simulink model "Just_The_Electrical_model"  (R2016a)
settings: Solver=VariableStepAuto  StartTime=0.0  StopTime=10.0  RelTol=1e-3
values from neighbouring files (symbols this model uses):
  BT = {}    [Electrical_model_settings.m]
  btc = {}    [Electrical_model_settings.m]
  col = {}    [Electrical_model_settings.m]
  elc = {}    [Electrical_model_settings.m]
  ess = {}    [Electrical_model_settings.m]
  fcc = {}    [Electrical_model_settings.m]
  flex = {}    [Electrical_model_settings.m]
  systemBase = {}    [Electrical_model_settings.m]
  wf = {}    [Electrical_model_settings.m]
  wt1 = {}    [Electrical_model_settings.m]
  wt2 = wt1    [Electrical_model_settings.m]
  wt3 = wt1    [Electrical_model_settings.m]
undefined symbols (not defined in the file or in its folder): avr, D1, Delta, DiscIntNeverNeededParam, f2ctrl, governor, interface, Lf1, sm, Ts, Ts_phy, Ts_sim, u0
libraries: powerlib x69, pwrsysBasic x68, simulink_extras x37, pwrsysVICtrl x22, powerlib_meascontrol x19, simulink x8, pwrsysVSrc x5, pwrsysTransf x5, pwrsys-matlab x1
(part 3 of 4)

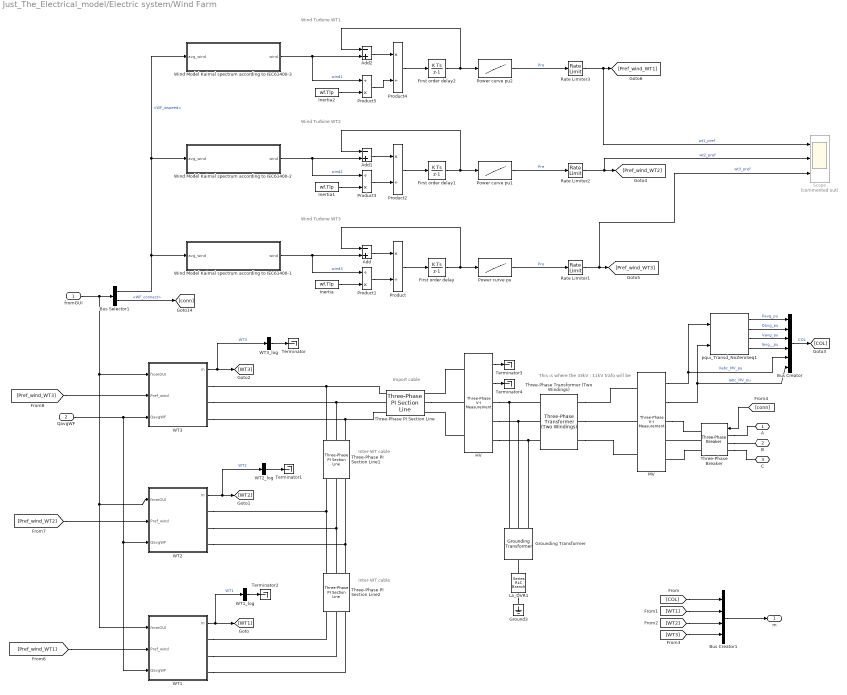
== system Just_The_Electrical_model/Electric system/Wind Farm ==
  note: Import cable
  note: This is where the 33kV : 11kV trafo will be
  note: Inter-WT cable
  note: Inter-WT cable
  note: Wind Turbine WT3
  note: Wind Turbine WT2
  note: Wind Turbine WT1
  fromGUI : Inport
  QavgWF : Inport  Port=2
  Add : Sum  Inputs=-+
  Add1 : Sum  Inputs=-+
  Add2 : Sum  Inputs=-+
  Bus Creator : BusCreator  Inputs=6
  Bus Creator1 : BusCreator  Inputs=4
  Bus Selector1 : BusSelector  OutputSignals=WF_wspeed,WF_connect
  First order delay : DiscreteIntegrator  gainval=1  SampleTime=Ts  ICPrevOutput=DiscIntNeverNeededParam  ICPrevScaledInput=DiscIntNeverNeededParam
  First order delay1 : DiscreteIntegrator  gainval=1  SampleTime=Ts  ICPrevOutput=DiscIntNeverNeededParam  ICPrevScaledInput=DiscIntNeverNeededParam
  First order delay2 : DiscreteIntegrator  gainval=1  SampleTime=Ts  ICPrevOutput=DiscIntNeverNeededParam  ICPrevScaledInput=DiscIntNeverNeededParam
  Ground3 : powerlib/Elements/Ground  LConnTagsString=a
  "Grounding Transformer " : powerlib/Elements/Grounding Transformer   UNITS=pu  NominalPower=[ col.Sn , systemBase.fn ]  NominalVoltage=systemBase.Vn  ZeroSequenceImpedance_pu=[0.025 0.75]  MagnetizationBranch_pu=[500 500]  ZeroSequenceImpedance_SI=[0.052083 589.05]  MagnetizationBranch_SI=[1041.7 3.927e+005]  Measurements=None
  HV : powerlib/Measurements/Three-Phase V-I Measurement  VoltageMeasurement=phase-to-ground  SetLabelV=off  LabelV=vgrid  Vpu=off  VpuLL=off  CurrentMeasurement=yes  SetLabelI=off  LabelI=igrid  Ipu=off  Pbase=sn  Vbase=uab  OutputType=Complex  PhasorSimulation=off  PSBequivalent=0
  Inertia : Constant  Value=wf.Tlp  SampleTime=-1
  Inertia1 : Constant  Value=wf.Tlp  SampleTime=-1
  Inertia2 : Constant  Value=wf.Tlp  SampleTime=-1
  La_DVR1 : powerlib/Elements/Series RLC Branch  LConnTagsString=__new0  RConnTagsString=__new0  BranchType=R  Resistance=250  Inductance=Lf1  SetiL0=off  InitialCurrent=0  Capacitance=1.0  Setx0=off  InitialVoltage=0  Measurements=None
  MV : powerlib/Measurements/Three-Phase V-I Measurement  VoltageMeasurement=phase-to-ground  SetLabelV=off  LabelV=vgrid  Vpu=off  VpuLL=off  CurrentMeasurement=yes  SetLabelI=off  LabelI=igrid  Ipu=off  Pbase=sn  Vbase=uab  OutputType=Complex  PhasorSimulation=off  PSBequivalent=0
  Power curve pu : Lookup  InputValues=wf.pcurve.wind  Table=wf.pcurve.power
  Power curve pu1 : Lookup  InputValues=wf.pcurve.wind  Table=wf.pcurve.power
  Power curve pu2 : Lookup  InputValues=wf.pcurve.wind  Table=wf.pcurve.power
  Product : Product  Inputs=*/
  Product1 : Product  Inputs=/*
  Product2 : Product  Inputs=*/
  Product3 : Product  Inputs=/*
  Product4 : Product  Inputs=*/
  Product5 : Product  Inputs=/*
  Rate Limiter1 : RateLimiter  RisingSlewLimit=100  FallingSlewLimit=-100  SampleTimeMode=inherited
  Rate Limiter2 : RateLimiter  RisingSlewLimit=100  FallingSlewLimit=-100  SampleTimeMode=inherited
  Rate Limiter3 : RateLimiter  RisingSlewLimit=100  FallingSlewLimit=-100  SampleTimeMode=inherited
  Scope : Scope  Commented=on  NumInputPorts=3
  Terminator{,1..4} (5 alike) : Terminator
  Three-Phase PI Section Line : powerlib/Elements/Three-Phase PI Section Line  LConnTagsString=a|b|c  RConnTagsString=A|B|C  Frequency=systemBase.fn  Resistances=[ col.Cable.Rpos col.Cable.Rzero]  Inductances=[ col.Cable.Lpos col.Cable.Lzero]  Capacitances=[col.Cable.Cpos col.Cable.Czero]  Length=col.Cable.Limport
  Three-Phase PI Section Line1 : powerlib/Elements/Three-Phase PI Section Line  LConnTagsString=a|b|c  RConnTagsString=A|B|C  Frequency=systemBase.fn  Resistances=[ col.Cable.Rpos col.Cable.Rzero]  Inductances=[ col.Cable.Lpos col.Cable.Lzero]  Capacitances=[col.Cable.Cpos col.Cable.Czero]  Length=col.Cable.LinterWT
  Three-Phase PI Section Line2 : powerlib/Elements/Three-Phase PI Section Line  LConnTagsString=a|b|c  RConnTagsString=A|B|C  Frequency=systemBase.fn  Resistances=[ col.Cable.Rpos col.Cable.Rzero]  Inductances=[ col.Cable.Lpos col.Cable.Lzero]  Capacitances=[col.Cable.Cpos col.Cable.Czero]  Length=col.Cable.LinterWT
  Three-Phase Transformer (Two Windings) : powerlib/Elements/Three-Phase Transformer (Two Windings)  Winding1Connection=Y  Winding2Connection=Delta (D1)  CoreType=Three-limb core (core-type)  SetSaturation=off  Hysteresis=off  DataFile='hysteresis'  SetInitialFlux=off  Measurements=None  UNITS=pu  NominalPower=[ col.Sn , systemBase.fn ]  Winding1=[ systemBase.Vn , col.Trafo.rsc/2 , col.Trafo.xsc/2 ]  Winding2=[ col.Un , col.Trafo.rsc/2 , col.Trafo.xsc/2 ]  Rm=500  Lm=500  L0=0.5  Saturation=[ 0,0 ; 0.0024,1.2 ; 1.0,1.52 ]  InitialFluxes=[0 0 0]  MoreParameters=off  BreakLoop=off  DataType=off  TransfoNumber=1
  Three-Phase Breaker : powerlib/Elements/Three-Phase Breaker  InitialState=closed  SwitchA=on  SwitchB=on  SwitchC=on  SwitchTimes="[1/60  5/60]"  External=on  BreakerResistance=0.01  SnubberResistance=1e6  SnubberCapacitance=1e9  Measurements=None
  WT1 : Subsystem
  WT1_log : BusSelector  OutputSignals=Pavg_pu,Qavg_pu,Vavg_pu,Vdc_pu,Idc_pu  OutputAsBus=on
  WT2 : Subsystem
  WT2_log : BusSelector  OutputSignals=Pavg_pu,Qavg_pu,Vavg_pu,Vdc_pu,Idc_pu  OutputAsBus=on
  WT3 : Subsystem
  WT3_log : BusSelector  OutputSignals=Pavg_pu,Qavg_pu,Vavg_pu,Vdc_pu,Idc_pu  OutputAsBus=on
  Wind Model Kaimal spectrum according to IEC61400-1 : Subsystem  TreatAsAtomicUnit=on  mask(Wind Model using Simulink Band-limited white noise generator){D_rotor=wf.Rdiam, L=wf.Lmm, turb_int=wf.Turb, T_sample=1/systemBase.fn, WhiteNoiseSeed=wt3.Kaimal.Seed}
      mask prompts: D_rotor "Rotor diameter [m]"; L "Length scale [m]"; turb_int "Turbulence intensity [%]"; T_sample "Sample time [sec]"; WhiteNoiseSeed "Kaimal white noise seed"
      mask help:
      | Implements a rotor wind model developped by RISOE National Laboratory based on Kaimal spectra. The model takes into account the rotational turbulences and the tower shadow.
      | This model uses the built-in band-limited white noise generator from Simulink
      mask init:
      | r = D_rotor/2;
      mask Display: disp('Wind\nModel')
  Wind Model Kaimal spectrum according to IEC61400-2 : Subsystem  TreatAsAtomicUnit=on  mask(Wind Model using Simulink Band-limited white noise generator){D_rotor=wf.Rdiam, L=wf.Lmm, turb_int=wf.Turb, T_sample=1/systemBase.fn, WhiteNoiseSeed=wt2.Kaimal.Seed}
      mask prompts: D_rotor "Rotor diameter [m]"; L "Length scale [m]"; turb_int "Turbulence intensity [%]"; T_sample "Sample time [sec]"; WhiteNoiseSeed "Kaimal white noise seed"
      mask help:
      | Implements a rotor wind model developped by RISOE National Laboratory based on Kaimal spectra. The model takes into account the rotational turbulences and the tower shadow.
      | This model uses the built-in band-limited white noise generator from Simulink
      mask init:
      | r = D_rotor/2;
      mask Display: disp('Wind\nModel')
  Wind Model Kaimal spectrum according to IEC61400-3 : Subsystem  TreatAsAtomicUnit=on  mask(Wind Model using Simulink Band-limited white noise generator){D_rotor=wf.Rdiam, L=wf.Lmm, turb_int=wf.Turb, T_sample=1/systemBase.fn, WhiteNoiseSeed=wt1.Kaimal.Seed}
      mask prompts: D_rotor "Rotor diameter [m]"; L "Length scale [m]"; turb_int "Turbulence intensity [%]"; T_sample "Sample time [sec]"; WhiteNoiseSeed "Kaimal white noise seed"
      mask help:
      | Implements a rotor wind model developped by RISOE National Laboratory based on Kaimal spectra. The model takes into account the rotational turbulences and the tower shadow.
      | This model uses the built-in band-limited white noise generator from Simulink
      mask init:
      | r = D_rotor/2;
      mask Display: disp('Wind\nModel')
  pqui_Transd_NoZeroSeq1 : pwrsysBasic/pqui_Transd_NoZeroSeq  Sn=col.Sn  Uanp=systemBase.Vn_phase*sqrt(2)  Iap=col.Iap*(col.Un/systemBase.Vn_phase)
  A : PMIOPort  Port=1  Side=Right
  B : PMIOPort  Port=2  Side=Right
  C : PMIOPort  Port=3  Side=Right
  m : Outport
  wires:
  [conn] -> Three-Phase Breaker/1
  MV/1 -> Bus Creator/5, pqui_Transd_NoZeroSeq1/1  "Vabc_MV_pu"
  HV/1 -> Terminator3/1
  HV/2 -> Terminator4/1
  MV/2 -> pqui_Transd_NoZeroSeq1/2, Bus Creator/6  "Iabc_MV_pu"
  pqui_Transd_NoZeroSeq1/1 -> Bus Creator/1  "Pavg_pu"
  pqui_Transd_NoZeroSeq1/4 -> Bus Creator/4  "Iavg__pu"
  pqui_Transd_NoZeroSeq1/2 -> Bus Creator/2  "Qavg_pu"
  pqui_Transd_NoZeroSeq1/3 -> Bus Creator/3  "Vavg_pu"
  Bus Creator/1 -> [COL]  "COL"
  WT3/1(m) -> WT3_log/1, [WT3]  "WT3"
  WT2/1(m) -> WT2_log/1, [WT2]  "WT2"
  Bus Creator1/1 -> m/1
  [COL] -> Bus Creator1/1
  [WT1] -> Bus Creator1/2
  [WT2] -> Bus Creator1/3
  [WT3] -> Bus Creator1/4
  WT3_log/1 -> Terminator/1
  WT2_log/1 -> Terminator1/1
  WT1/1(m) -> WT1_log/1, [WT1]  "WT1"
  WT1_log/1 -> Terminator2/1
  fromGUI/1 -> WT1/1(fromGUI), WT2/1(fromGUI), WT3/1(fromGUI), Bus Selector1/1
  Bus Selector1/2 -> [conn]  "<WF_connect>"
  Product/1 -> First order delay/1
  Add/1 -> Product/1
  Wind Model Kaimal spectrum according to IEC61400-1/1(wind) -> Product1/1, Add/2  "wind3"
  Inertia/1 -> Product1/2
  Product1/1 -> Product/2
  First order delay/1 -> Power curve pu/1, Add/1
  Bus Selector1/1 -> Wind Model Kaimal spectrum according to IEC61400-3/1(avg_wind), Wind Model Kaimal spectrum according to IEC61400-2/1(avg_wind), Wind Model Kaimal spectrum according to IEC61400-1/1(avg_wind)  "<WF_wspeed>"
  Power curve pu/1 -> Rate Limiter1/1  "Pre"
  Rate Limiter1/1 -> Scope/3, [Pref_wind_WT3]  "wt3_pref"
  [Pref_wind_WT3] -> WT3/2(Pref_wind)
  Product2/1 -> First order delay1/1
  Add1/1 -> Product2/1
  Wind Model Kaimal spectrum according to IEC61400-2/1(wind) -> Product3/1, Add1/2  "wind2"
  Inertia1/1 -> Product3/2
  Product3/1 -> Product2/2
  First order delay1/1 -> Power curve pu1/1, Add1/1
  Power curve pu1/1 -> Rate Limiter2/1  "Pre"
  Rate Limiter2/1 -> Scope/2, [Pref_wind_WT2]  "wt2_pref"
  Product4/1 -> First order delay2/1
  Add2/1 -> Product4/1
  Wind Model Kaimal spectrum according to IEC61400-3/1(wind) -> Product5/1, Add2/2  "wind1"
  Inertia2/1 -> Product5/2
  Product5/1 -> Product4/2
  First order delay2/1 -> Power curve pu2/1, Add2/1
  Power curve pu2/1 -> Rate Limiter3/1  "Pre"
  Rate Limiter3/1 -> Scope/1, [Pref_wind_WT1]  "wt1_pref"
  [Pref_wind_WT1] -> WT1/2(Pref_wind)
  [Pref_wind_WT2] -> WT2/2(Pref_wind)
  QavgWF/1 -> WT1/3(QavgWF), WT2/3(QavgWF), WT3/3(QavgWF)
  connections:
  Three-Phase Breaker/RConn3 -- MV/RConn3
  Three-Phase Transformer (Two Windings)/LConn3 -- MV/LConn3
  Three-Phase Transformer (Two Windings)/LConn1 -- MV/LConn1
  Three-Phase Transformer (Two Windings)/LConn2 -- MV/LConn2
  MV/RConn1 -- Three-Phase Breaker/RConn1
  Three-Phase PI Section Line/RConn2 -- HV/LConn2
  Three-Phase Breaker/RConn2 -- MV/RConn2
  HV/LConn1 -- Three-Phase PI Section Line/RConn1
  HV/LConn3 -- Three-Phase PI Section Line/RConn3
  Three-Phase Breaker/LConn2 -- B/RConn1
  Three-Phase PI Section Line1/LConn3 -- WT3/RConn3 -- Three-Phase PI Section Line/LConn3
  Three-Phase Breaker/LConn1 -- A/RConn1
  Three-Phase Breaker/LConn3 -- C/RConn1
  Three-Phase PI Section Line1/LConn2 -- WT3/RConn2 -- Three-Phase PI Section Line/LConn2
  Three-Phase PI Section Line/LConn1 -- WT3/RConn1 -- Three-Phase PI Section Line1/LConn1
  Three-Phase PI Section Line2/LConn1 -- WT2/RConn1 -- Three-Phase PI Section Line1/RConn1
  Three-Phase PI Section Line2/LConn2 -- WT2/RConn2 -- Three-Phase PI Section Line1/RConn2
  Three-Phase PI Section Line2/LConn3 -- WT2/RConn3 -- Three-Phase PI Section Line1/RConn3
  WT1/RConn1 -- Three-Phase PI Section Line2/RConn1
  WT1/RConn2 -- Three-Phase PI Section Line2/RConn2
  WT1/RConn3 -- Three-Phase PI Section Line2/RConn3
  HV/RConn1 -- "Grounding Transformer "/LConn3 -- Three-Phase Transformer (Two Windings)/RConn1
  HV/RConn2 -- "Grounding Transformer "/LConn2 -- Three-Phase Transformer (Two Windings)/RConn2
  HV/RConn3 -- "Grounding Transformer "/LConn1 -- Three-Phase Transformer (Two Windings)/RConn3
  La_DVR1/RConn1 -- "Grounding Transformer "/RConn1
  La_DVR1/LConn1 -- Ground3/LConn1

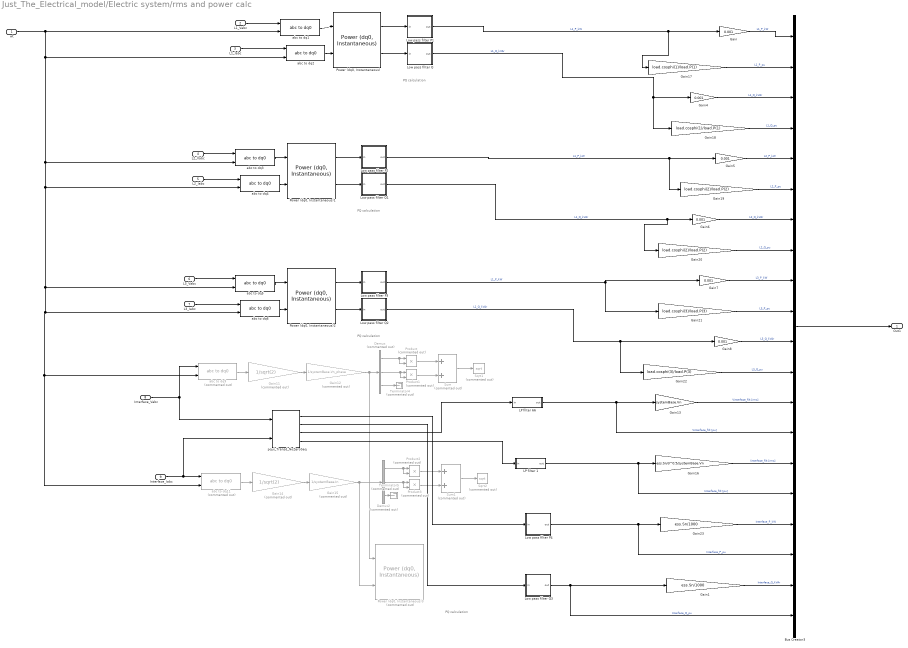
== system Just_The_Electrical_model/Electric system/rms and power calc ==
  note: PQ calculation
  note: PQ calculation
  note: PQ calculation
  note: PQ calculation
  wt : Inport
  L1_Vabc : Inport  Port=2
  L1_Iabc : Inport  Port=3
  L2_Vabc : Inport  Port=4
  L2_Iabc : Inport  Port=5
  L3_Vabc : Inport  Port=6
  L3_Iabc : Inport  Port=7
  Interface_Vabc : Inport  Port=8
  Interface_Iabc : Inport  Port=9
  Bus Creator3 : BusCreator  Inputs=20
  Demux : Demux  Commented=on  Outputs=3
  Demux2 : Demux  Commented=on  Outputs=3
  Gain{,4..8} (6 alike) : Gain  Gain=0.001
  Gain1 : Gain  Gain=ess.Sn/1000
  Gain11 : Gain  Commented=on  Gain=1/sqrt(2)
  Gain12 : Gain  Commented=on  Gain=1/systemBase.Vn_phase
  Gain13 : Gain  Gain=systemBase.Vn
  Gain14 : Gain  Commented=on  Gain=1/sqrt(2)
  Gain15 : Gain  Commented=on  Gain=1/systemBase.In
  Gain16 : Gain  Gain=ess.Sn/3^0.5/systemBase.Vn
  Gain17 : Gain  Gain=load.cosphi(1)/load.P(1)
  Gain18 : Gain  Gain=load.cosphi(1)/load.P(1)
  Gain19 : Gain  Gain=load.cosphi(2)/load.P(2)
  Gain20 : Gain  Gain=load.cosphi(2)/load.P(2)
  Gain21 : Gain  Gain=load.cosphi(3)/load.P(3)
  Gain22 : Gain  Gain=load.cosphi(3)/load.P(3)
  Gain23 : Gain  Gain=ess.Sn/1000
  LP filter 1 : Subsystem  mask(Discrete first order low pass filter){tau=sm.V_measure_T, Ts=Ts, x0=avr.init, y0=avr.init}
      mask prompts: tau "Filter time constant [s]"; Ts "Sampling time [s]"; x0 "Initial input"; y0 "Initial output"
      mask help: Discrete first order low pass filter derived from a continous filter by bilinear transformation.
  LP filter 66 : Subsystem  mask(Discrete first order low pass filter){tau=sm.V_measure_T, Ts=Ts, x0=avr.init, y0=avr.init}
      mask prompts: tau "Filter time constant [s]"; Ts "Sampling time [s]"; x0 "Initial input"; y0 "Initial output"
      mask help: Discrete first order low pass filter derived from a continous filter by bilinear transformation.
  Low pass filter P1 : Subsystem  mask(Discrete first order low pass filter){tau=sm.P_measure, Ts=Ts, x0=0, y0=0}
      mask prompts: tau "Filter time constant [s]"; Ts "Sampling time [s]"; x0 "Initial input"; y0 "Initial output"
      mask help: Discrete first order low pass filter derived from a continous filter by bilinear transformation.
  Low pass filter P2 : Subsystem  mask(Discrete first order low pass filter){tau=sm.P_measure, Ts=Ts, x0=0, y0=0}
      mask prompts: tau "Filter time constant [s]"; Ts "Sampling time [s]"; x0 "Initial input"; y0 "Initial output"
      mask help: Discrete first order low pass filter derived from a continous filter by bilinear transformation.
  Low pass filter P3 : Subsystem  mask(Discrete first order low pass filter){tau=sm.P_measure, Ts=Ts, x0=0, y0=0}
      mask prompts: tau "Filter time constant [s]"; Ts "Sampling time [s]"; x0 "Initial input"; y0 "Initial output"
      mask help: Discrete first order low pass filter derived from a continous filter by bilinear transformation.
  Low pass filter P4 : Subsystem  mask(Discrete first order low pass filter){tau=sm.P_measure, Ts=Ts, x0=0, y0=0}
      mask prompts: tau "Filter time constant [s]"; Ts "Sampling time [s]"; x0 "Initial input"; y0 "Initial output"
      mask help: Discrete first order low pass filter derived from a continous filter by bilinear transformation.
  Low pass filter Q : Subsystem  mask(Discrete first order low pass filter){tau=sm.Q_measure, Ts=Ts, x0=0, y0=0}
      mask prompts: tau "Filter time constant [s]"; Ts "Sampling time [s]"; x0 "Initial input"; y0 "Initial output"
      mask help: Discrete first order low pass filter derived from a continous filter by bilinear transformation.
  Low pass filter Q1 : Subsystem  mask(Discrete first order low pass filter){tau=sm.Q_measure, Ts=Ts, x0=0, y0=0}
      mask prompts: tau "Filter time constant [s]"; Ts "Sampling time [s]"; x0 "Initial input"; y0 "Initial output"
      mask help: Discrete first order low pass filter derived from a continous filter by bilinear transformation.
  Low pass filter Q2 : Subsystem  mask(Discrete first order low pass filter){tau=sm.Q_measure, Ts=Ts, x0=0, y0=0}
      mask prompts: tau "Filter time constant [s]"; Ts "Sampling time [s]"; x0 "Initial input"; y0 "Initial output"
      mask help: Discrete first order low pass filter derived from a continous filter by bilinear transformation.
  Low pass filter Q3 : Subsystem  mask(Discrete first order low pass filter){tau=sm.Q_measure, Ts=Ts, x0=0, y0=0}
      mask prompts: tau "Filter time constant [s]"; Ts "Sampling time [s]"; x0 "Initial input"; y0 "Initial output"
      mask help: Discrete first order low pass filter derived from a continous filter by bilinear transformation.
  "Power (dq0, Instantaneous)" : powerlib_meascontrol/Measurements/Power (dq0, Instantaneous)
  "Power (dq0, Instantaneous)1" : powerlib_meascontrol/Measurements/Power (dq0, Instantaneous)
  "Power (dq0, Instantaneous)2" : powerlib_meascontrol/Measurements/Power (dq0, Instantaneous)
  "Power (dq0, Instantaneous)3" : powerlib_meascontrol/Measurements/Power (dq0, Instantaneous)  Commented=on
  Product{,1..3} (4 alike) : Product  Commented=on
  Sqrt1 : Sqrt  Commented=on  SaturateOnIntegerOverflow=on
  Sqrt2 : Sqrt  Commented=on  SaturateOnIntegerOverflow=on
  Sum : Sum  Commented=on
  Sum1 : Sum  Commented=on
  Terminator4 : Terminator  Commented=on
  Terminator5 : Terminator  Commented=on
  abc to dq{1..6} (6 alike) : powerlib_meascontrol/Transformations/abc to dq0  Alignment=Aligned with phase A axis
  abc to dq11 : powerlib_meascontrol/Transformations/abc to dq0  Commented=on  Alignment=Aligned with phase A axis
  abc to dq9 : powerlib_meascontrol/Transformations/abc to dq0  Commented=on  Alignment=Aligned with phase A axis
  pqui_Transd_NoZeroSeq : pwrsysBasic/pqui_Transd_NoZeroSeq  Sn=ess.Sn  Uanp=systemBase.Vn*(2/3)^0.5  Iap=ess.Iap*(ess.Un/systemBase.Vn)
  Out1 : Outport
  wires:
  "Power (dq0, Instantaneous)"/1 -> Low pass filter P1/1(in)
  Gain22/1 -> Bus Creator3/12  "L3_Q_pu"
  Low pass filter Q3/1(out) -> Gain1/1, Bus Creator3/20  "Interface_Q_pu"
  Gain19/1 -> Bus Creator3/6  "L2_P_pu"
  Gain5/1 -> Bus Creator3/5  "L2_P_kW"
  Gain18/1 -> Bus Creator3/4  "L1_Q_pu"
  Gain4/1 -> Bus Creator3/3  "L1_Q_kVAr"
  Gain17/1 -> Bus Creator3/2  "L1_P_pu"
  wt/1 -> abc to dq1/2, abc to dq2/2, abc to dq3/2, abc to dq4/2, abc to dq5/2, abc to dq11/2, abc to dq9/2, abc to dq6/2
  Interface_Iabc/1 -> pqui_Transd_NoZeroSeq/2, abc to dq11/1
  abc to dq11/1 -> Gain14/1
  Gain21/1 -> Bus Creator3/10  "L3_P_pu"
  Low pass filter P4/1(out) -> Bus Creator3/18, Gain23/1  "Interface_P_pu"
  Gain20/1 -> Bus Creator3/8  "L2_Q_pu"
  Gain1/1 -> Bus Creator3/19  "Interface_Q_kVAr"
  LP filter 1/1(out) -> Bus Creator3/16, Gain16/1  "Iinterface_filt [pu]"
  Interface_Vabc/1 -> abc to dq9/1, pqui_Transd_NoZeroSeq/1
  Low pass filter Q2/1(out) -> Gain22/1, Gain8/1  "L1_Q_kVAr"
  Low pass filter P3/1(out) -> Gain7/1, Gain21/1  "L1_P_kW"
  abc to dq9/1 -> Gain11/1
  Gain16/1 -> Bus Creator3/15  "Iinterfase_filt [rms]"
  Product2/1 -> Sum1/1
  Demux2/1 -> Product2/1, Product2/2
  LP filter 66/1(out) -> Bus Creator3/14, Gain13/1  "Vinterface_filt [pu]"
  Product/1 -> Sum/1
  Gain11/1 -> Gain12/1
  Gain23/1 -> Bus Creator3/17  "Interface_P_kW"
  Sum/1 -> Sqrt1/1
  Gain15/1 -> Demux2/1, "Power (dq0, Instantaneous)3"/2
  Gain12/1 -> Demux/1, "Power (dq0, Instantaneous)3"/1
  Product3/1 -> Sum1/2
  Product1/1 -> Sum/2
  Demux/1 -> Product/1, Product/2
  Gain14/1 -> Gain15/1
  Demux2/2 -> Product3/1, Product3/2
  Gain13/1 -> Bus Creator3/13  "Vinterfase_filt [rms]"
  Sum1/1 -> Sqrt2/1
  Demux/2 -> Product1/1, Product1/2
  "Power (dq0, Instantaneous)1"/1 -> Low pass filter P2/1(in)
  Gain8/1 -> Bus Creator3/11  "L3_Q_kVAr"
  L3_Vabc/1 -> abc to dq5/1
  L2_Iabc/1 -> abc to dq4/1
  L2_Vabc/1 -> abc to dq3/1
  abc to dq3/1 -> "Power (dq0, Instantaneous)1"/1
  Gain7/1 -> Bus Creator3/9  "L3_P_kW"
  L3_Iabc/1 -> abc to dq6/1
  "Power (dq0, Instantaneous)2"/1 -> Low pass filter P3/1(in)
  Low pass filter Q/1(out) -> Gain4/1, Gain18/1  "L1_Q_kVAr"
  "Power (dq0, Instantaneous)1"/2 -> Low pass filter Q1/1(in)
  "Power (dq0, Instantaneous)2"/2 -> Low pass filter Q2/1(in)
  abc to dq4/1 -> "Power (dq0, Instantaneous)1"/2
  Low pass filter P1/1(out) -> Gain/1, Gain17/1  "L1_P_kW"
  abc to dq5/1 -> "Power (dq0, Instantaneous)2"/1
  Low pass filter Q1/1(out) -> Gain6/1, Gain20/1  "L1_Q_kVAr"
  Bus Creator3/1 -> Out1/1
  abc to dq6/1 -> "Power (dq0, Instantaneous)2"/2
  Low pass filter P2/1(out) -> Gain5/1, Gain19/1  "L1_P_kW"
  Gain6/1 -> Bus Creator3/7  "L2_Q_kVAr"
  L1_Iabc/1 -> abc to dq2/1
  L1_Vabc/1 -> abc to dq1/1
  abc to dq2/1 -> "Power (dq0, Instantaneous)"/2
  abc to dq1/1 -> "Power (dq0, Instantaneous)"/1
  Gain/1 -> Bus Creator3/1  "L1_P_kW"
  "Power (dq0, Instantaneous)"/2 -> Low pass filter Q/1(in)
  Demux2/3 -> Terminator5/1
  Demux/3 -> Terminator4/1
  pqui_Transd_NoZeroSeq/3 -> LP filter 66/1(in)
  pqui_Transd_NoZeroSeq/4 -> LP filter 1/1(in)
  pqui_Transd_NoZeroSeq/1 -> Low pass filter P4/1(in)
  pqui_Transd_NoZeroSeq/2 -> Low pass filter Q3/1(in)

== system Just_The_Electrical_model/Electric system/Automatic voltage regulator/LP filter active power ==
  in : Inport
  Discrete Transfer Fcn (with initial outputs) : simulink_extras/Additional Discrete/Discrete Transfer Fcn (with initial outputs)  N=[1/tau*Ts/2 1/tau*Ts/2]  D=[(1/tau*Ts/2+1) (1/tau*Ts/2-1)]  U0=x0  Y0=y0  TS=Ts
  out : Outport
  wires:
  in/1 -> Discrete Transfer Fcn (with initial outputs)/1
  Discrete Transfer Fcn (with initial outputs)/1 -> out/1

== system Just_The_Electrical_model/Electric system/Automatic voltage regulator/LP filter frequency ==
  in : Inport
  Discrete Transfer Fcn (with initial outputs) : simulink_extras/Additional Discrete/Discrete Transfer Fcn (with initial outputs)  N=[1/tau*Ts/2 1/tau*Ts/2]  D=[(1/tau*Ts/2+1) (1/tau*Ts/2-1)]  U0=x0  Y0=y0  TS=Ts
  out : Outport
  wires:
  Discrete Transfer Fcn (with initial outputs)/1 -> out/1
  in/1 -> Discrete Transfer Fcn (with initial outputs)/1

== system Just_The_Electrical_model/Electric system/Automatic voltage regulator/LP filter frequency1 ==
  in : Inport
  Discrete Transfer Fcn (with initial outputs) : simulink_extras/Additional Discrete/Discrete Transfer Fcn (with initial outputs)  N=[1/tau*Ts/2 1/tau*Ts/2]  D=[(1/tau*Ts/2+1) (1/tau*Ts/2-1)]  U0=x0  Y0=y0  TS=Ts
  out : Outport
  wires:
  Discrete Transfer Fcn (with initial outputs)/1 -> out/1
  in/1 -> Discrete Transfer Fcn (with initial outputs)/1

== system Just_The_Electrical_model/Electric system/Automatic voltage regulator/LP filter frequency2 ==
  in : Inport
  Discrete Transfer Fcn (with initial outputs) : simulink_extras/Additional Discrete/Discrete Transfer Fcn (with initial outputs)  N=[1/tau*Ts/2 1/tau*Ts/2]  D=[(1/tau*Ts/2+1) (1/tau*Ts/2-1)]  U0=x0  Y0=y0  TS=Ts
  out : Outport
  wires:
  Discrete Transfer Fcn (with initial outputs)/1 -> out/1
  in/1 -> Discrete Transfer Fcn (with initial outputs)/1

== system Just_The_Electrical_model/Electric system/Automatic voltage regulator/LP filter reactive power ==
  in : Inport
  Discrete Transfer Fcn (with initial outputs) : simulink_extras/Additional Discrete/Discrete Transfer Fcn (with initial outputs)  N=[1/tau*Ts/2 1/tau*Ts/2]  D=[(1/tau*Ts/2+1) (1/tau*Ts/2-1)]  U0=x0  Y0=y0  TS=Ts
  out : Outport
  wires:
  Discrete Transfer Fcn (with initial outputs)/1 -> out/1
  in/1 -> Discrete Transfer Fcn (with initial outputs)/1

== system Just_The_Electrical_model/Electric system/Automatic voltage regulator/PID_Governor1 ==
  in : Inport
  reset_int : Inport  Port=2
  reset_value : Inport  Port=3
  Discrete Derivative : simulink/Discrete/Discrete Derivative  gainval=1.0  ICPrevScaledInput=0.0  InputProcessing=Inherited  OutMin=[]  OutMax=[]  OutDataType=fixdt(1, 16)  OutScaling=2^-10  DoSatur=off
  Discrete-Time Integrator : DiscreteIntegrator  IntegratorMethod=Integration: Trapezoidal  ExternalReset=level  InitialConditionSource=external  InitialCondition=xi  InitialConditionSetting=State (most efficient)  SampleTime=Ts  LimitOutput=on  UpperSaturationLimit=up_sat_limit  LowerSaturationLimit=low_sat_limit  ICPrevOutput=DiscIntNeverNeededParam  ICPrevScaledInput=DiscIntNeverNeededParam
  Integral Gain : Gain  DisableCoverage=on  Gain=ki
  Integral Gain1 : Gain  DisableCoverage=on  Gain=kd
  LP filter power : Subsystem  mask(Discrete first order low pass filter){tau=governor.derivativeLP, Ts=Ts, x0=0, y0=0}
      mask prompts: tau "Filter time constant [s]"; Ts "Sampling time [s]"; x0 "Initial input"; y0 "Initial output"
      mask help: Discrete first order low pass filter derived from a continous filter by bilinear transformation.
  P+I : Sum  Inputs=+++
  Proportional Gain : Gain  DisableCoverage=on  Gain=kp
  Saturation : Saturate  UpperLimit=up_sat_limit  LowerLimit=low_sat_limit
  out : Outport
  wires:
  LP filter power/1(out) -> Discrete Derivative/1
  Discrete Derivative/1 -> P+I/3
  Integral Gain1/1 -> LP filter power/1(in)
  reset_value/1 -> Discrete-Time Integrator/3
  reset_int/1 -> Discrete-Time Integrator/2
  Saturation/1 -> out/1
  Proportional Gain/1 -> P+I/1
  in/1 -> Integral Gain/1, Integral Gain1/1, Proportional Gain/1
  P+I/1 -> Saturation/1
  Integral Gain/1 -> Discrete-Time Integrator/1
  Discrete-Time Integrator/1 -> P+I/2

== system Just_The_Electrical_model/Electric system/Automatic voltage regulator/guiPushButtonInterface ==
  In1 : Inport
  Data Type Conversion6 : DataTypeConversion  OutDataTypeStr=double  RndMeth=Round
  Detect Change : simulink/Logic and Bit Operations/Detect Change  vinit=0  InputProcessing=Inherited  OutDataTypeStr=boolean
  IC1 : InitialCondition  Value=0
  Out1 : Outport
  wires:
  IC1/1 -> Out1/1
  Data Type Conversion6/1 -> IC1/1
  Detect Change/1 -> Data Type Conversion6/1
  In1/1 -> Detect Change/1

== system Just_The_Electrical_model/Electric system/DC Grid/DC-Link Model ==
  FC_Idc : Inport
  ELY_Idc : Inport  Port=2
  Batt_Idc : Inport  Port=3
  EGSTON_Vdc : Inport  Port=4
  ESSsim_Vdc : Inport  Port=5
  EGSTON_enable : Inport  Port=6
  Digital first order LPF1 : pwrsysBasic/Digital first order LPF  Ts=Ts  fcutout=ess.Fsw/10
  Digital first order LPF3 : pwrsysBasic/Digital first order LPF  Ts=Ts  fcutout=ess.Fsw/10
  Gain1 : Gain  Gain=ess.Udc
  Saturation1 : Saturate  UpperLimit=2*ess.Udc  LowerLimit=0.50*ess.Udc
  Sum : Sum  Inputs=3
  Switch EGSTON : Switch  Criteria=u2 > Threshold
  DCL_Idc : Outport
  DCL_Vdc : Outport  Port=2
  wires:
  Digital first order LPF3/1 -> DCL_Idc/1  "DCL_Idc"
  FC_Idc/1 -> Sum/1  "FC_idc"
  ELY_Idc/1 -> Sum/2  "ELY_idc"
  Batt_Idc/1 -> Sum/3  "Batt_idc"
  Digital first order LPF1/1 -> DCL_Vdc/1  "DCL_Vdc"
  Sum/1 -> Digital first order LPF3/1
  EGSTON_Vdc/1 -> Switch EGSTON/1
  Switch EGSTON/1 -> Saturation1/1
  ESSsim_Vdc/1 -> Gain1/1
  EGSTON_enable/1 -> Switch EGSTON/2
  Gain1/1 -> Switch EGSTON/3
  Saturation1/1 -> Digital first order LPF1/1

== system Just_The_Electrical_model/Electric system/DC Grid/guiPushButtonInterface ==
  In1 : Inport
  Data Type Conversion6 : DataTypeConversion  OutDataTypeStr=double  RndMeth=Round
  Detect Change : simulink/Logic and Bit Operations/Detect Change  vinit=0  InputProcessing=Inherited  OutDataTypeStr=boolean
  IC1 : InitialCondition  Value=0
  Out1 : Outport
  wires:
  IC1/1 -> Out1/1
  Data Type Conversion6/1 -> IC1/1
  Detect Change/1 -> Data Type Conversion6/1
  In1/1 -> Detect Change/1

== system Just_The_Electrical_model/Electric system/Power Management System/guiPushButtonInterface ==
  In1 : Inport
  Data Type Conversion6 : DataTypeConversion  OutDataTypeStr=double  RndMeth=Round
  Detect Change : simulink/Logic and Bit Operations/Detect Change  vinit=0  InputProcessing=Inherited  OutDataTypeStr=boolean
  IC1 : InitialCondition  Value=0
  Out1 : Outport
  wires:
  IC1/1 -> Out1/1
  Data Type Conversion6/1 -> IC1/1
  Detect Change/1 -> Data Type Conversion6/1
  In1/1 -> Detect Change/1

== system Just_The_Electrical_model/Electric system/Rotation1/guiPushButtonInterface ==
  In1 : Inport
  Data Type Conversion6 : DataTypeConversion  OutDataTypeStr=double  RndMeth=Round
  Detect Change : simulink/Logic and Bit Operations/Detect Change  vinit=0  InputProcessing=Inherited  OutDataTypeStr=boolean
  IC1 : InitialCondition  Value=0
  Out1 : Outport
  wires:
  IC1/1 -> Out1/1
  Data Type Conversion6/1 -> IC1/1
  Detect Change/1 -> Data Type Conversion6/1
  In1/1 -> Detect Change/1

== system Just_The_Electrical_model/Electric system/SM_simple/LP filter  ==
  in : Inport
  Discrete Transfer Fcn (with initial outputs) : simulink_extras/Additional Discrete/Discrete Transfer Fcn (with initial outputs)  N=[1/tau*Ts/2 1/tau*Ts/2]  D=[(1/tau*Ts/2+1) (1/tau*Ts/2-1)]  U0=x0  Y0=y0  TS=Ts
  out : Outport
  wires:
  Discrete Transfer Fcn (with initial outputs)/1 -> out/1
  in/1 -> Discrete Transfer Fcn (with initial outputs)/1

== system Just_The_Electrical_model/Electric system/SM_simple/LP filter 1 ==
  in : Inport
  Discrete Transfer Fcn (with initial outputs) : simulink_extras/Additional Discrete/Discrete Transfer Fcn (with initial outputs)  N=[1/tau*Ts/2 1/tau*Ts/2]  D=[(1/tau*Ts/2+1) (1/tau*Ts/2-1)]  U0=x0  Y0=y0  TS=Ts
  out : Outport
  wires:
  Discrete Transfer Fcn (with initial outputs)/1 -> out/1
  in/1 -> Discrete Transfer Fcn (with initial outputs)/1

== system Just_The_Electrical_model/Electric system/SM_simple/LP filter 2 ==
  in : Inport
  Discrete Transfer Fcn (with initial outputs) : simulink_extras/Additional Discrete/Discrete Transfer Fcn (with initial outputs)  N=[1/tau*Ts/2 1/tau*Ts/2]  D=[(1/tau*Ts/2+1) (1/tau*Ts/2-1)]  U0=x0  Y0=y0  TS=Ts
  out : Outport
  wires:
  in/1 -> Discrete Transfer Fcn (with initial outputs)/1
  Discrete Transfer Fcn (with initial outputs)/1 -> out/1

== system Just_The_Electrical_model/Electric system/SM_simple/LP filter 3 ==
  in : Inport
  Discrete Transfer Fcn (with initial outputs) : simulink_extras/Additional Discrete/Discrete Transfer Fcn (with initial outputs)  N=[1/tau*Ts/2 1/tau*Ts/2]  D=[(1/tau*Ts/2+1) (1/tau*Ts/2-1)]  U0=x0  Y0=y0  TS=Ts
  out : Outport
  wires:
  in/1 -> Discrete Transfer Fcn (with initial outputs)/1
  Discrete Transfer Fcn (with initial outputs)/1 -> out/1

== system Just_The_Electrical_model/Electric system/SM_simple/LP filter 3  ==
  in : Inport
  Discrete Transfer Fcn (with initial outputs) : simulink_extras/Additional Discrete/Discrete Transfer Fcn (with initial outputs)  N=[1/tau*Ts/2 1/tau*Ts/2]  D=[(1/tau*Ts/2+1) (1/tau*Ts/2-1)]  U0=x0  Y0=y0  TS=Ts
  out : Outport
  wires:
  Discrete Transfer Fcn (with initial outputs)/1 -> out/1
  in/1 -> Discrete Transfer Fcn (with initial outputs)/1

== system Just_The_Electrical_model/Electric system/SM_simple/LP filter 3 1 ==
  in : Inport
  Discrete Transfer Fcn (with initial outputs) : simulink_extras/Additional Discrete/Discrete Transfer Fcn (with initial outputs)  N=[1/tau*Ts/2 1/tau*Ts/2]  D=[(1/tau*Ts/2+1) (1/tau*Ts/2-1)]  U0=x0  Y0=y0  TS=Ts
  out : Outport
  wires:
  Discrete Transfer Fcn (with initial outputs)/1 -> out/1
  in/1 -> Discrete Transfer Fcn (with initial outputs)/1

== system Just_The_Electrical_model/Electric system/SM_simple/LP filter 3 2 ==
  in : Inport
  Discrete Transfer Fcn (with initial outputs) : simulink_extras/Additional Discrete/Discrete Transfer Fcn (with initial outputs)  N=[1/tau*Ts/2 1/tau*Ts/2]  D=[(1/tau*Ts/2+1) (1/tau*Ts/2-1)]  U0=x0  Y0=y0  TS=Ts
  out : Outport
  wires:
  Discrete Transfer Fcn (with initial outputs)/1 -> out/1
  in/1 -> Discrete Transfer Fcn (with initial outputs)/1

== system Just_The_Electrical_model/Electric system/SM_simple/LP filter 4 ==
  in : Inport
  Discrete Transfer Fcn (with initial outputs) : simulink_extras/Additional Discrete/Discrete Transfer Fcn (with initial outputs)  N=[1/tau*Ts/2 1/tau*Ts/2]  D=[(1/tau*Ts/2+1) (1/tau*Ts/2-1)]  U0=x0  Y0=y0  TS=Ts
  out : Outport
  wires:
  Discrete Transfer Fcn (with initial outputs)/1 -> out/1
  in/1 -> Discrete Transfer Fcn (with initial outputs)/1

== system Just_The_Electrical_model/Electric system/SM_simple/LP filter 5 ==
  in : Inport
  Discrete Transfer Fcn (with initial outputs) : simulink_extras/Additional Discrete/Discrete Transfer Fcn (with initial outputs)  N=[1/tau*Ts/2 1/tau*Ts/2]  D=[(1/tau*Ts/2+1) (1/tau*Ts/2-1)]  U0=x0  Y0=y0  TS=Ts
  out : Outport
  wires:
  Discrete Transfer Fcn (with initial outputs)/1 -> out/1
  in/1 -> Discrete Transfer Fcn (with initial outputs)/1

== system Just_The_Electrical_model/Electric system/SM_simple/LP filter 6 ==
  in : Inport
  Discrete Transfer Fcn (with initial outputs) : simulink_extras/Additional Discrete/Discrete Transfer Fcn (with initial outputs)  N=[1/tau*Ts/2 1/tau*Ts/2]  D=[(1/tau*Ts/2+1) (1/tau*Ts/2-1)]  U0=x0  Y0=y0  TS=Ts
  out : Outport
  wires:
  in/1 -> Discrete Transfer Fcn (with initial outputs)/1
  Discrete Transfer Fcn (with initial outputs)/1 -> out/1

== system Just_The_Electrical_model/Electric system/SM_simple/LP filter 66 ==
  in : Inport
  Discrete Transfer Fcn (with initial outputs) : simulink_extras/Additional Discrete/Discrete Transfer Fcn (with initial outputs)  N=[1/tau*Ts/2 1/tau*Ts/2]  D=[(1/tau*Ts/2+1) (1/tau*Ts/2-1)]  U0=x0  Y0=y0  TS=Ts
  out : Outport
  wires:
  Discrete Transfer Fcn (with initial outputs)/1 -> out/1
  in/1 -> Discrete Transfer Fcn (with initial outputs)/1

== system Just_The_Electrical_model/Electric system/SM_simple/LP filter 67 ==
  in : Inport
  Discrete Transfer Fcn (with initial outputs) : simulink_extras/Additional Discrete/Discrete Transfer Fcn (with initial outputs)  N=[1/tau*Ts/2 1/tau*Ts/2]  D=[(1/tau*Ts/2+1) (1/tau*Ts/2-1)]  U0=x0  Y0=y0  TS=Ts
  out : Outport
  wires:
  Discrete Transfer Fcn (with initial outputs)/1 -> out/1
  in/1 -> Discrete Transfer Fcn (with initial outputs)/1

== system Just_The_Electrical_model/Electric system/SM_simple/Low pass filter P1 ==
  in : Inport
  Discrete Transfer Fcn (with initial outputs) : simulink_extras/Additional Discrete/Discrete Transfer Fcn (with initial outputs)  N=[1/tau*Ts/2 1/tau*Ts/2]  D=[(1/tau*Ts/2+1) (1/tau*Ts/2-1)]  U0=x0  Y0=y0  TS=Ts
  out : Outport
  wires:
  Discrete Transfer Fcn (with initial outputs)/1 -> out/1
  in/1 -> Discrete Transfer Fcn (with initial outputs)/1

== system Just_The_Electrical_model/Electric system/SM_simple/Low pass filter Q ==
  in : Inport
  Discrete Transfer Fcn (with initial outputs) : simulink_extras/Additional Discrete/Discrete Transfer Fcn (with initial outputs)  N=[1/tau*Ts/2 1/tau*Ts/2]  D=[(1/tau*Ts/2+1) (1/tau*Ts/2-1)]  U0=x0  Y0=y0  TS=Ts
  out : Outport
  wires:
  Discrete Transfer Fcn (with initial outputs)/1 -> out/1
  in/1 -> Discrete Transfer Fcn (with initial outputs)/1

== system Just_The_Electrical_model/Electric system/SM_simple/powerCalcAndFilt1 ==
  note: Low pass filter power measurement
  Vabc : Inport
  Iabc : Inport  Port=2
  LP filter frequency1 : Subsystem  mask(Discrete first order low pass filter){tau=sm.P_measure, Ts=Ts, x0=avr.init, y0=avr.init}
      mask prompts: tau "Filter time constant [s]"; Ts "Sampling time [s]"; x0 "Initial input"; y0 "Initial output"
      mask help: Discrete first order low pass filter derived from a continous filter by bilinear transformation.
  LP filter frequency2 : Subsystem  mask(Discrete first order low pass filter){tau=sm.Q_measure, Ts=Ts, x0=avr.init, y0=avr.init}
      mask prompts: tau "Filter time constant [s]"; Ts "Sampling time [s]"; x0 "Initial input"; y0 "Initial output"
      mask help: Discrete first order low pass filter derived from a continous filter by bilinear transformation.
  "Power (3ph, Instantaneous)1" : powerlib_meascontrol/Measurements/Power (3ph, Instantaneous)
  P_filt : Outport
  Q_filt1 : Outport  Port=2
  wires:
  LP filter frequency2/1(out) -> Q_filt1/1
  LP filter frequency1/1(out) -> P_filt/1
  "Power (3ph, Instantaneous)1"/2 -> LP filter frequency2/1(in)
  Iabc/1 -> "Power (3ph, Instantaneous)1"/2
  Vabc/1 -> "Power (3ph, Instantaneous)1"/1
  "Power (3ph, Instantaneous)1"/1 -> LP filter frequency1/1(in)

== system Just_The_Electrical_model/Electric system/SM_simple/sinusRefGen ==
  note: Models the voltage dependency of speed. Asume linear dependency
  GenBackEmf [VrmsLL] : Inport
  freq Hz : Inport  Port=2
  phase (rad) : Inport  Port=3
  deltaAmplitudeIndividual : Inport  Port=4
  phaseSkiftIndividual : Inport  Port=5
  Constant1 : Constant  Value=2*pi()/3
  Constant2 : Constant  Value=2*pi()
  Constant3 : Constant  Value=2*pi()/3
  Constant4 : Constant
  Constant5 : Constant  Value=pi()
  Discrete-Time Integrator : DiscreteIntegrator  InitialConditionSetting=State (most efficient)  SampleTime=-1  ICPrevOutput=DiscIntNeverNeededParam  ICPrevScaledInput=DiscIntNeverNeededParam
  Divide : Product  Inputs=*/
  Gain1 : Gain  Gain=sqrt(2)/sqrt(3)
  Gain3 : Gain
  Product{,1..4} (5 alike) : Product
  Rated Freq : Constant  Value=sm.fn
  Sum1 : Sum  Inputs=|+-
  Sum2 : Sum  Inputs=|++
  Sum3 : Sum  Inputs=+++
  Trigonometric Function : Trigonometry
  Trigonometric Function1 : Trigonometry
  Trigonometric Function2 : Trigonometry
  a : Outport
  b : Outport  Port=2
  c : Outport  Port=3
  wires:
  Constant5/1 -> Sum3/1
  Constant4/1 -> Product4/1
  phaseSkiftIndividual/1 -> ?
  deltaAmplitudeIndividual/1 -> ?
  Product4/1 -> Product1/2, Product2/2, Product3/2
  Trigonometric Function2/1 -> Product3/1
  Discrete-Time Integrator/1 -> Sum3/2
  Divide/1 -> Gain3/1
  Rated Freq/1 -> Divide/2
  Constant2/1 -> Product/2
  Trigonometric Function1/1 -> Product2/1
  Product1/1 -> a/1
  Product3/1 -> c/1
  Gain1/1 -> Product4/2
  Product2/1 -> b/1
  GenBackEmf [VrmsLL]/1 -> Gain1/1
  Constant3/1 -> Sum2/2
  Constant1/1 -> Sum1/2
  Sum2/1 -> Trigonometric Function2/1
  Sum1/1 -> Trigonometric Function1/1
  Trigonometric Function/1 -> Product1/1
  Sum3/1 -> Sum2/1, Sum1/1, Trigonometric Function/1
  phase (rad)/1 -> Sum3/3
  Product/1 -> Discrete-Time Integrator/1
  freq Hz/1 -> Product/1, Divide/1

== system Just_The_Electrical_model/Electric system/Turbine Governor1/LP filter power ==
  in : Inport
  Discrete Transfer Fcn (with initial outputs) : simulink_extras/Additional Discrete/Discrete Transfer Fcn (with initial outputs)  N=[1/tau*Ts/2 1/tau*Ts/2]  D=[(1/tau*Ts/2+1) (1/tau*Ts/2-1)]  U0=x0  Y0=y0  TS=Ts
  out : Outport
  wires:
  Discrete Transfer Fcn (with initial outputs)/1 -> out/1
  in/1 -> Discrete Transfer Fcn (with initial outputs)/1

== system Just_The_Electrical_model/Electric system/Turbine Governor1/LP filter power2 ==
  in : Inport
  Discrete Transfer Fcn (with initial outputs) : simulink_extras/Additional Discrete/Discrete Transfer Fcn (with initial outputs)  N=[1/tau*Ts/2 1/tau*Ts/2]  D=[(1/tau*Ts/2+1) (1/tau*Ts/2-1)]  U0=x0  Y0=y0  TS=Ts
  out : Outport
  wires:
  Discrete Transfer Fcn (with initial outputs)/1 -> out/1
  in/1 -> Discrete Transfer Fcn (with initial outputs)/1
